simulink model "lab7_inciso1"  (R2021a)
settings: Solver=VariableStepAuto  StartTime=0.0  StopTime=F  RelTol=1e-3
values from neighbouring files (symbols this model uses):
  Acl = A3-B3*K    [Lab7.m]
  B3 = [1/(r1*c1);0;0]    [Lab7.m]
  C3 = [0,1,0]    [Lab7.m]
  Nbar = rscale(sys,K)    [Lab7.m]
  T = 1/0.667    (= 1.49925037481)    [Lab7.m]
settings Model: Creator=fersa  LastModifiedBy=fersa

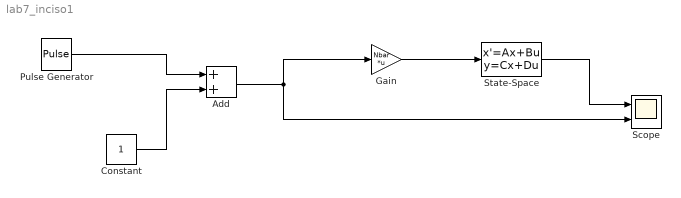
== system lab7_inciso1 ==
  Add : Sum
  Constant : Constant
  Gain : Gain  Gain=Nbar  Multiplication=Matrix(K*u) (u vector)
  Pulse Generator : DiscretePulseGenerator  PulseType=Time based  Period=T  PulseWidth=50  PhaseDelay=0.75
  Scope : Scope  NumInputPorts=2
  State-Space : StateSpace  A=Acl  B=B3  C=C3  D=0  InitialCondition=0  ParameterTunability=Unconstrained
  wires:
  Gain/1 -> State-Space/1
  State-Space/1 -> Scope/1
  Pulse Generator/1 -> Add/1
  Constant/1 -> Add/2
  Add/1 -> Gain/1, Scope/2
